simulink model "main"  (Simulink 4.00)
settings: Solver=ode45  StartTime=0.0  StopTime=10.0  RelTol=1e-3
settings Model: LastModifiedBy=User

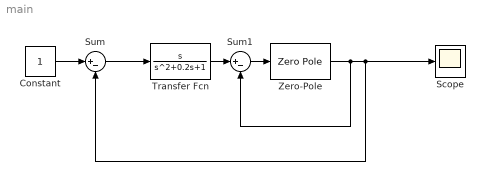
== system main ==
  Constant : Constant  Value=1
  Scope : Scope
      settings: TimeRange=auto  YMin=-5  YMax=5  SaveToWorkspace=off  SaveName=ScopeData  LimitDataPoints=on  MaxDataPoints=5000
  Sum : Sum  Inputs=|+-  SaturateOnIntegerOverflow=on
  Sum1 : Sum  Inputs=|+-  SaturateOnIntegerOverflow=on
  Transfer Fcn : TransferFcn  Numerator=[1 0]  Denominator=[1 0.2 1]  AbsoluteTolerance=auto  Realization=auto
  Zero-Pole : ZeroPole  Zeros=[0]  Poles=[-0.03 -1]  Gain=[1]  AbsoluteTolerance=auto
  wires:
  Constant/1 -> Sum/1
  Sum/1 -> Transfer Fcn/1
  Transfer Fcn/1 -> Sum1/1
  Sum1/1 -> Zero-Pole/1
  Zero-Pole/1 -> Sum1/2, Scope/1, Sum/2
